simulink model "lm35sensor_Task"  (R2018b)
settings: Solver=FixedStepAuto  StartTime=0.0  StopTime=inf  RelTol=1e-3  EnableMultiTasking=on
libraries: arduinolib x2
settings Model: SimulationMode=external  ExtModeTrigDuration=2  Creator=DELL  LastModifiedBy=DELL
settings OptimizationCC: EnhancedBackFolding=on  PassReuseOutputArgsAs=Individual arguments  MaxStackSize=64  OptimizeBlockOrder=speed  DifferentSizesBufferReuse=on  OptimizationCustomize=off
settings DebuggingCC: ParameterTunabilityLossMsg=error
settings HardwareCC: ProdBitPerInt=16  ProdBitPerPointer=16  ProdBitPerSizeT=16  ProdBitPerPtrDiffT=16  ProdLargestAtomicFloat=None  ProdWordSize=8  ProdHWDeviceType=Atmel->AVR
settings SFSimCC: MATLABDynamicMemAlloc=off
settings RTWCC: SystemTargetFile=ert.tlc  HardwareBoard=Arduino Uno  TemplateMakefile=ert_default_tmf  GenerateReport=on  Toolchain=Arduino AVR  BuildConfiguration=Faster Runs  IncludeHyperlinkInReport=on  LaunchReport=on  GenerateTraceInfo=on  GenerateTraceReport=on  GenerateTraceReportSl=on  GenerateTraceReportSf=on  GenerateTraceReportEml=on
settings CodeAppCC: ForceParamTrailComments=on  IgnoreCustomStorageClasses=off  OperatorAnnotations=on  SimulinkDataObjDesc=on  SFDataObjDesc=on  InsertBlockDesc=on
settings ERTTargetCC: SupportContinuousTime=on  SupportVariableSizeSignals=on

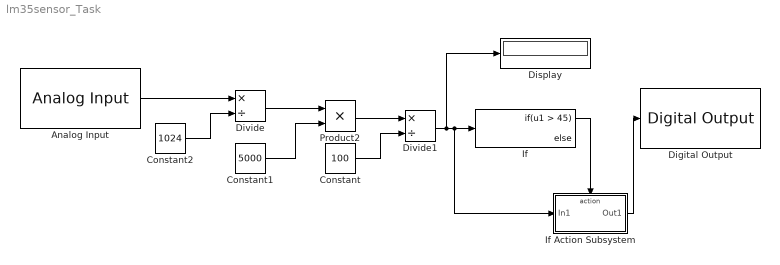
== system lm35sensor_Task ==
  Analog Input : arduinolib/Analog Input  pinNumber=4  ReadResultsOnly=off  ConversionTriggerSource=Software  ExternalTriggerType=uint32(0)  OutputDataType=uint16  EnableConversionCompleteNotify=off  EnableOuputStatus=off  SampleTime=1  blockPlatform=arduino
  Constant : Constant  Value=100
  Constant1 : Constant  Value=5000
  Constant2 : Constant  Value=1024
  Digital Output : arduinolib/Digital Output  pinNumber=9  blockPlatform=arduino
  Display : Display
  Divide : Product  Inputs=*/
  Divide1 : Product  Inputs=*/
  If : If  IfExpression=u1 > 45
  If Action Subsystem : Subsystem  TreatAsAtomicUnit=on
  Product2 : Product
  wires:
  Analog Input/1 -> Divide/1
  Constant2/1 -> Divide/2
  Divide/1 -> Product2/1
  Constant1/1 -> Product2/2
  Product2/1 -> Divide1/1
  Constant/1 -> Divide1/2
  Divide1/1 -> Display/1, If Action Subsystem/1(In1), If/1
  If/1 -> If Action Subsystem/Action
  If Action Subsystem/1(Out1) -> Digital Output/1

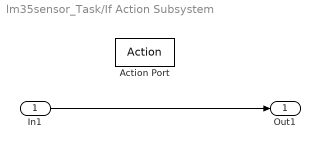
== system lm35sensor_Task/If Action Subsystem ==
  In1 : Inport
  Action Port : ActionPort  ActionType=then
  Out1 : Outport
  wires:
  In1/1 -> Out1/1
